simulink model "stop_ex"  (R2020a)
settings: Solver=FixedStepDiscrete  StartTime=0.0  StopTime=100  FixedStep=1  RelTol=1e-3
settings Model: Creator=lenovo  LastModifiedBy=DELL
settings DataIOCC: ReturnWorkspaceOutputs=off
settings DebuggingCC: ArithmeticOperatorsInVariantConditions=warning
settings SFSimCC: SimUseLocalCustomCode=off  CustomCodeUndefinedFunction=UseInterfaceOnly
settings RTWCC: RTWUseLocalCustomCode=off

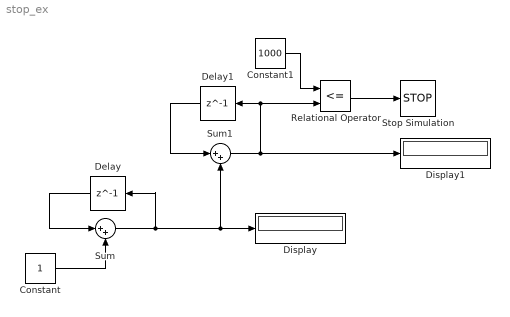
== system stop_ex ==
  Constant : Constant
  Constant1 : Constant  Value=1000
  Delay : Delay  DelayLength=1  InitialCondition=0
  Delay1 : Delay  DelayLength=1  InitialCondition=0
  Display : Display
  Display1 : Display
  Relational Operator : RelationalOperator  Operator=<=  OutDataTypeStr=boolean  RndMeth=Simplest
  Stop Simulation : Stop
  Sum : Sum  Inputs=|++
  Sum1 : Sum  Inputs=|++
  wires:
  Constant/1 -> Sum/2
  Sum/1 -> Display/1, Sum1/2, Delay/1
  Delay/1 -> Sum/1
  Sum1/1 -> Display1/1, Relational Operator/2, Delay1/1
  Delay1/1 -> Sum1/1
  Relational Operator/1 -> Stop Simulation/1
  Constant1/1 -> Relational Operator/1
